simulink model "block_diagram_simplified"  (Simulink 6.3)
settings: Solver=ode23  StartTime=0.0  StopTime=5  FixedStep=0.0001  RelTol=1e-9  AbsTol=1e-11
values from neighbouring files (symbols this model uses):
  b_op = damping_vec(b)    [automated_bode.m]    (also in find_tf.m = 1000000000; parameters.m = 100; parameters2.m = 20)
  b_spring = spring_damping_vec(b_sp)    [automated_bode.m]    (also in parameters.m = 0.01; parameters2.m = 100)
  bit_offset = 128    [parameters2.m]
  freq = frequency_vec(i)    [automated_bode.m]    (also in parameters.m = 100; parameters2.m = 1)
  J_T = 1.25E-3 / n / n    (= 9.96492346939e-08)    [analytical_bode_comparing.m]    (also in analytical_bode_creator.m; find_tf.m; parameters.m; parameters2.m)
  K_ampl = 10    [analytical_bode_comparing.m]    (also in parameters.m; parameters2.m)
  K_emf = 3.29E-3 / 60    (= 5.48333333333e-05)    [analytical_bode_comparing.m]    (also in analytical_bode_creator.m; find_tf.m; parameters.m; parameters2.m)
  k_eq = spring_stiffness_vec(k)    [analytical_bode_comparing.m]    (also in analytical_bode_creator.m = 6; find_tf.m = 6; parameters.m = 6000; parameters2.m = 6000)
  k_op = stiffness_vec(k)    [automated_bode.m]    (also in find_tf.m = 1000000000; parameters.m = 100; parameters2.m = 200)
  K_PID2Vardu = 1/51    (= 0.0196078431373)    [analytical_bode_comparing.m]    (also in parameters2.m)
  K_tau = efficiency*31.4E-3    (= 0.01884)    [analytical_bode_comparing.m]    (also in analytical_bode_creator.m = 0.0314; find_tf.m = 0.0314; parameters.m = 0.0314; parameters2.m = 0.0314)
  K_V2dist = -1    [find_tf.m]    (also in parameters2.m = -0.00036)
  L_a = 5.8E-3    (= 0.0058)    [analytical_bode_comparing.m]    (also in analytical_bode_creator.m; find_tf.m; parameters.m; parameters2.m)
  L_CL = 20E-3    (= 0.02)    [analytical_bode_comparing.m]    (also in analytical_bode_creator.m; calc_JTOT.m; find_tf.m; parameters.m)
  m_2 = 7E-3    (= 0.007)    [analytical_bode_comparing.m]    (also in analytical_bode_creator.m; find_tf.m; parameters.m; parameters2.m)
  n = 112    [analytical_bode_comparing.m]    (also in analytical_bode_creator.m; calc_JTOT.m; find_tf.m; parameters.m)
  R_a = 118.6    [analytical_bode_comparing.m]    (also in analytical_bode_creator.m; find_tf.m; parameters.m; parameters2.m)
  um_gain = -1000000    [analytical_bode_comparing.m]    (also in parameters2.m)
  V_offset = -20    [parameters.m]    (also in parameters2.m = -25)
libraries: simulink_extras x1
settings Model: LastModifiedBy=oechslin

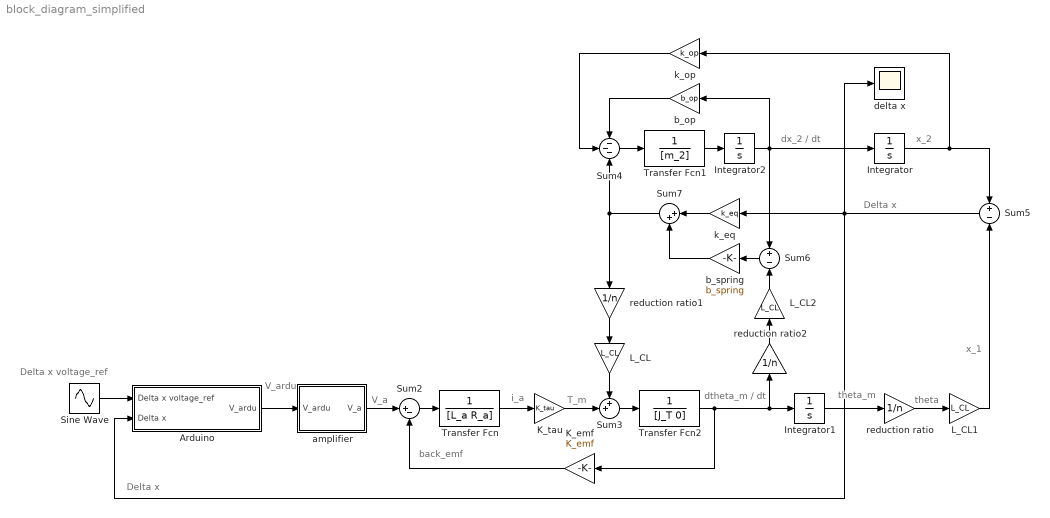
== system block_diagram_simplified ==
  note: Delta x voltage_ref
  note: x_2
  note: Delta x
  note: x_1
  note: dtheta_m / dt
  note: theta_m
  note: back_emf
  note: V_a
  note: V_ardu
  note: Delta x
  note: theta
  note: dx_2 / dt
  note: i_a
  note: T_m
  Arduino : Subsystem
  Integrator : Integrator
  Integrator1 : Integrator
  Integrator2 : Integrator
  K_emf : Gain  Orientation=left  Gain=K_emf
  K_tau : Gain  Gain=K_tau
  L_CL : Gain  Orientation=down  Gain=L_CL
  L_CL1 : Gain  Gain=L_CL
  L_CL2 : Gain  Orientation=up  Gain=L_CL
  Sine Wave : Sin  Amplitude=0.3  Bias=0.35  Frequency=freq * 2*3.1416  SampleTime=0
  Sum2 : Sum  Inputs=|+-
  Sum3 : Sum  Inputs=++|
  Sum4 : Sum  Inputs=---
  Sum5 : Sum  Orientation=left  Inputs=+|-
  Sum6 : Sum  Orientation=left  Inputs=+|-
  Sum7 : Sum  Orientation=left  Inputs=|++
  Transfer Fcn : TransferFcn  Denominator=[L_a R_a]
  Transfer Fcn1 : TransferFcn  Denominator=[m_2]
  Transfer Fcn2 : TransferFcn  Denominator=[J_T 0]
  "amplifier " : Subsystem
  b_op : Gain  Orientation=left  Gain=b_op
  b_spring : Gain  Orientation=left  Gain=b_spring
  delta x : Scope
      settings: TimeRange=10
  k_eq : Gain  Orientation=left  Gain=k_eq
  k_op : Gain  Orientation=left  Gain=k_op
  reduction ratio : Gain  Gain=1/n
  reduction ratio1 : Gain  Orientation=down  Gain=1/n
  reduction ratio2 : Gain  Orientation=up  Gain=1/n
  wires:
  Arduino/1(V_ardu) -> "amplifier "/1(V_ardu)
  "amplifier "/1(V_a) -> Sum2/1
  Sum2/1 -> Transfer Fcn/1
  Transfer Fcn/1 -> K_tau/1
  L_CL/1 -> Sum3/1
  K_tau/1 -> Sum3/2
  Sum4/1 -> Transfer Fcn1/1
  Integrator/1 -> k_op/1, Sum5/1
  Sum5/1 -> Arduino/2(Delta x), delta x/1, k_eq/1
  L_CL1/1 -> Sum5/2
  Integrator1/1 -> reduction ratio/1
  Transfer Fcn2/1 -> Integrator1/1, reduction ratio2/1, K_emf/1
  Sum3/1 -> Transfer Fcn2/1
  K_emf/1 -> Sum2/2
  Sine Wave/1 -> Arduino/1(Delta x voltage_ref)
  reduction ratio/1 -> L_CL1/1
  L_CL2/1 -> Sum6/2
  Sum6/1 -> b_spring/1
  b_spring/1 -> Sum7/2
  k_eq/1 -> Sum7/1
  Sum7/1 -> Sum4/3, reduction ratio1/1
  Transfer Fcn1/1 -> Integrator2/1
  reduction ratio2/1 -> L_CL2/1
  reduction ratio1/1 -> L_CL/1
  k_op/1 -> Sum4/2
  b_op/1 -> Sum4/1
  Integrator2/1 -> Integrator/1, Sum6/1, b_op/1

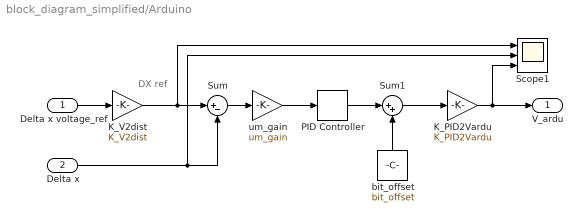
== system block_diagram_simplified/Arduino ==
  note: DX ref
  Delta x voltage_ref : Inport
  Delta x : Inport  Port=2
  K_PID2Vardu : Gain  Gain=K_PID2Vardu
  K_V2dist : Gain  Gain=K_V2dist
  PID Controller : simulink_extras/Additional Linear/PID Controller  P=0.2  I=0  D=0
  Scope1 : Scope  NumInputPorts=3
      settings: TimeRange=5  YMin=-4.06576e-020~-0.0003~-2.5  YMax=0.00075~0~0  SaveName=ScopeData2
  Sum : Sum  Inputs=|+-
  Sum1 : Sum  Inputs=|++
  bit_offset : Constant  Orientation=up  Value=bit_offset
  um_gain : Gain  Gain=um_gain
  V_ardu : Outport
  wires:
  Delta x voltage_ref/1 -> K_V2dist/1
  Sum/1 -> um_gain/1
  K_V2dist/1 -> Sum/1, Scope1/1
  Delta x/1 -> Sum/2, Scope1/2
  PID Controller/1 -> Sum1/1
  um_gain/1 -> PID Controller/1
  K_PID2Vardu/1 -> V_ardu/1, Scope1/3
  Sum1/1 -> K_PID2Vardu/1
  bit_offset/1 -> Sum1/2

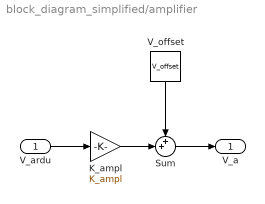
== system block_diagram_simplified/amplifier  ==
  V_ardu : Inport
  K_ampl : Gain  Gain=K_ampl
  Sum : Sum  Inputs=++|
  V_offset : Constant  Orientation=down  Value=V_offset
  V_a : Outport
  wires:
  V_offset/1 -> Sum/1
  V_ardu/1 -> K_ampl/1
  K_ampl/1 -> Sum/2
  Sum/1 -> V_a/1
